simulink model "septic_new"  (R2015a)
settings: Solver=ode45  StartTime=0.0  StopTime=0.1  RelTol=1e-3
undefined symbols (not defined in the file): Ion, Lithium
libraries: powerlib x19, electricdrivelib x1, simulink x1, powerlib_meascontrol x1
settings Model: Creator=HP  LastModifiedBy=HP

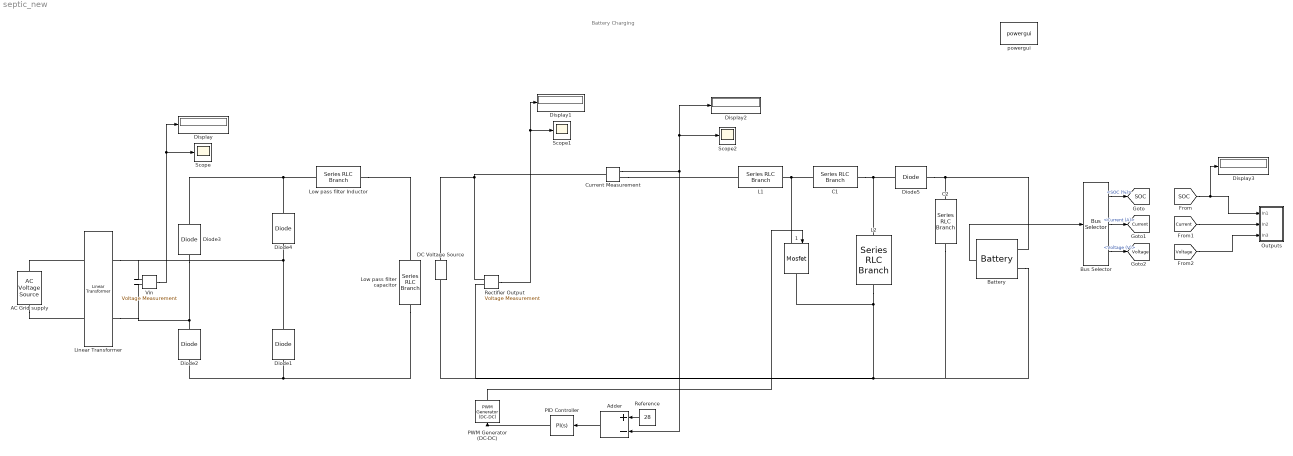
== system septic_new ==
  note: Battery Charging
  1 : powerlib/Power Electronics/Mosfet  Ron=0.1  Lon=0  Rd=0.01  Vfd=0  IC=0  Rs=1e5  Cs=inf  Measurements=off
  AC Grid supply : powerlib/Electrical Sources/AC Voltage Source  Amplitude=325.26  Phase=0  Frequency=50  SampleTime=0  Measurements=None
  Adder : Sum  Inputs=+-
  Battery : electricdrivelib/Extra Sources/Battery  BatType=Lithium-Ion  ShowDetailedParameters=off  NomV=48  NomQ=28  SOC=0  PresetModel=on  MaxQ=28  FullV=55.8714  Dis_rate=12.1739  R=0.017143  Normal_OP=25.3217  expZone="[51.8585      1.37565]"  current=[6.5 13 32.5]  Units=Time  Batt_Tr=30
  Bus Selector : BusSelector  OutputSignals=SOC (%),Current (A),Voltage (V)
  C1 : powerlib/Elements/Series RLC Branch  LConnTagsString=__new0  RConnTagsString=__new0  BranchType=C  Resistance=1  Inductance=28.57e-6  SetiL0=off  InitialCurrent=0  Capacitance=4700e-6  Setx0=off  InitialVoltage=0  Measurements=None
  C2 : powerlib/Elements/Series RLC Branch  LConnTagsString=__new0  RConnTagsString=__new0  BranchType=C  Resistance=1  Inductance=28.57e-6  SetiL0=off  InitialCurrent=0  Capacitance=4700e-6  Setx0=off  InitialVoltage=0  Measurements=None
  Current Measurement : powerlib/Measurements/Current Measurement  PhasorSimulation=off  OutputType=Complex  PSBequivalent=0
  DC Voltage Source : powerlib/Electrical Sources/DC Voltage Source  Amplitude=30  Measurements=None
  Diode{1..5} (5 alike) : powerlib/Power Electronics/Diode  Ron=0.001  Lon=0  Vf=0.8  IC=0  UseSnubber=off  Rs=500  Cs=250e-9  Measurements=off
  Display{,1..3} (4 alike) : Display
      Display3 settings: Decimation=2
  L1 : powerlib/Elements/Series RLC Branch  LConnTagsString=__new0  RConnTagsString=__new0  BranchType=L  Resistance=1  Inductance=10e-4  SetiL0=off  InitialCurrent=0  Capacitance=1e-6  Setx0=off  InitialVoltage=0  Measurements=None
  L2 : powerlib/Elements/Series RLC Branch  LConnTagsString=__new0  RConnTagsString=__new0  BranchType=L  Resistance=1  Inductance=10e-4  SetiL0=off  InitialCurrent=0  Capacitance=1e-6  Setx0=off  InitialVoltage=0  Measurements=None
  Linear Transformer : powerlib/Elements/Linear Transformer  UNITS=SI  NominalPower=[ 1e3 50 ]  winding1=[10 0 0]  winding2=[1 0 0]  ThreeWindings=off  winding3=[3.15e+05 0.7938 0.084225]  RmLm=[inf inf]  Measurements=None  DataType=on
  Low pass filter Inductor : powerlib/Elements/Series RLC Branch  LConnTagsString=__new0  RConnTagsString=__new0  BranchType=L  Resistance=1  Inductance=1e-3  SetiL0=off  InitialCurrent=0  Capacitance=1e-6  Setx0=off  InitialVoltage=0  Measurements=None
  Low pass filter capacitor : powerlib/Elements/Series RLC Branch  LConnTagsString=__new0  RConnTagsString=__new0  BranchType=C  Resistance=1000  Inductance=1e-3  SetiL0=off  InitialCurrent=0  Capacitance=4700e-6  Setx0=off  InitialVoltage=0  Measurements=None
  Outputs : Subsystem
  PID Controller : simulink/Continuous/PID Controller  Controller=PI  TimeDomain=Continuous-time  SampleTime=-1  IntegratorMethod=Forward Euler  FilterMethod=Forward Euler  Form=Parallel  UseFilter=on  ControllerParametersSource=internal  P=10  I=1  D=0.15  N=100  InitialConditionSource=internal  InitialConditionForIntegrator=0  InitialConditionForFilter=0  ExternalReset=none  LimitOutput=on  UpperSaturationLimit=0.9  LowerSaturationLimit=0  LinearizeAsGain=on  AntiWindupMode=clamping  Kb=1  TrackingMode=off  Kt=1  PParamMin=[]  PParamMax=[]  IParamMin=[]  IParamMax=[]  DParamMin=[]  DParamMax=[]  NParamMin=[]  NParamMax=[]  KbParamMin=[]  KbParamMax=[]  KtParamMin=[]  KtParamMax=[]  POutMin=[]  POutMax=[]  IOutMin=[]  IOutMax=[]  DOutMin=[]  DOutMax=[]  NOutMin=[]  NOutMax=[]  KbOutMin=[]  KbOutMax=[]  KtOutMin=[]  KtOutMax=[]  IntegratorOutMin=[]  IntegratorOutMax=[]  FilterOutMin=[]  FilterOutMax=[]  SumOutMin=[]  SumOutMax=[]  SumI1OutMin=[]  SumI1OutMax=[]  SumI2OutMin=[]  SumI2OutMax=[]  SumI3OutMin=[]  SumI3OutMax=[]  SumDOutMin=[]  SumDOutMax=[]  SaturationOutMin=[]  SaturationOutMax=[]  IntegratorContinuousStateAttributes=''  IntegratorStateMustResolveToSignalObject=off  IntegratorRTWStateStorageClass=Auto  FilterContinuousStateAttributes=''  FilterStateMustResolveToSignalObject=off  FilterRTWStateStorageClass=Auto  DifferentiatorICPrevScaledInput=0  DifferentiatorOutMin=[]  DifferentiatorOutMax=[]
  PWM Generator (DC-DC) : powerlib_meascontrol/Pulse & Signal Generators/PWM Generator (DC-DC)  Fsw=30000  Ts=5e-6
  Rectifier Output : powerlib/Measurements/Voltage Measurement  PhasorSimulation=off  OutputType=Complex  PSBequivalent=0
  Reference : Constant  Value=28
  Scope : Scope
      settings: YMin=-50  YMax=50  SaveName=ScopeData2
  Scope1 : Scope
      settings: YMin=200  YMax=250  SaveName=ScopeData3
  Scope2 : Scope
      settings: TimeRange=0.1  YMin=30  YMax=33  SaveName=ScopeData4
  Vin : powerlib/Measurements/Voltage Measurement  PhasorSimulation=off  OutputType=Complex  PSBequivalent=0
  powergui : powerlib/powergui  Priority=1  SimulationMode=Continuous  SolverType=Tustin/Backward Euler (TBE)  SampleTime=5e-6  frequency=60  SPID=off  DisableSnubberDevices=off  DisableRonSwitches=off  DisableVfSwitches=off  SwTol=0  DisplayEquations=off  Interpol=off  methode=off  Ts=100  FunctionMessages=off  echomessages=off  HookPort=off  EnableUseOfTLC=off  x0status=blocks  frequencyindice=0  Pbase=100e6  ErrMax=1e-4  Iterations=50  UnitsV=kV  UnitsW=MW  buscounter=0  RestoreLinks=warning  ResistiveCurrentMeasurement=off  Frange=[0:2:500]  Ylog=off  Xlog=on  ShowGrid=off  save=off  variable=ZData  structure=0  ZoomFFT=off  StartTime=0.0  cycles=1  DisplayStyle=1  fundamental=60  FreqAxis=off  MaxFrequency=1000  frequencyindicesteady=1  RmsSteady=1  display=off
  tag scope: Current=global, SOC=global, Voltage=global
  wires:
  Battery/1 -> Bus Selector/1
  Bus Selector/3 -> [Voltage]  "<Voltage (V)>"
  Bus Selector/2 -> [Current]  "<Current (A)>"
  Bus Selector/1 -> [SOC]  "<SOC (%)>"
  PWM Generator (DC-DC)/1 -> 1/1
  PID Controller/1 -> PWM Generator (DC-DC)/1
  Adder/1 -> PID Controller/1
  [Current] -> Outputs/2(In2)
  [SOC] -> Display3/1, Outputs/1(In1)
  [Voltage] -> Outputs/3(In3)
  Vin/1 -> Scope/1, Display/1
  Rectifier Output/1 -> Scope1/1, Display1/1
  Current Measurement/1 -> Display2/1, Scope2/1, Adder/2
  Reference/1 -> Adder/1
  connections:
  L1/RConn1 -- C1/LConn1 -- 1/LConn1
  C1/RConn1 -- Diode5/LConn1 -- L2/LConn1
  Linear Transformer/RConn2 -- Vin/LConn2 -- Diode3/LConn1 -- Diode2/RConn1
  Linear Transformer/RConn1 -- Vin/LConn1 -- Diode1/RConn1 -- Diode4/LConn1
  Diode3/RConn1 -- Low pass filter Inductor/LConn1 -- Diode4/RConn1
  Linear Transformer/LConn1 -- AC Grid supply/RConn1
  AC Grid supply/LConn1 -- Linear Transformer/LConn2
  Diode5/RConn1 -- C2/LConn1 -- Battery/LConn1
  Rectifier Output/LConn1 -- DC Voltage Source/RConn1 -- Current Measurement/LConn1
  Current Measurement/RConn1 -- L1/LConn1
  L2/RConn1 -- 1/RConn1 -- DC Voltage Source/LConn1 -- Rectifier Output/LConn2 -- C2/RConn1 -- Battery/LConn2
  Low pass filter Inductor/RConn1 -- Low pass filter capacitor/LConn1
  Low pass filter capacitor/RConn1 -- Diode2/LConn1 -- Diode1/LConn1

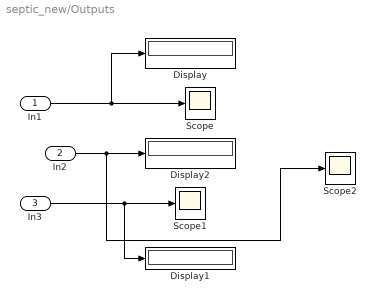
== system septic_new/Outputs ==
  In1 : Inport
  In2 : Inport  Port=2
  In3 : Inport  Port=3
  Display : Display
      settings: Decimation=2
  Display1 : Display
      settings: Decimation=2
  Display2 : Display
      settings: Decimation=2
  Scope : Scope
      settings: YMin=50  YMax=70
  Scope1 : Scope
      settings: YMin=-0  YMax=100
  Scope2 : Scope
      settings: YMin=-100  YMax=0  SaveName=ScopeData5
  wires:
  In3/1 -> Display1/1, Scope1/1
  In1/1 -> Display/1, Scope/1
  In2/1 -> Scope2/1, Display2/1
